simulink model "cooling_system"  (R2025b)
settings: Solver=ode4  StartTime=0.0  StopTime=200  FixedStep=0.1  RelTol=1e-3
libraries: simulink x14
settings Model: Creator=srija  LastModifiedBy=srija

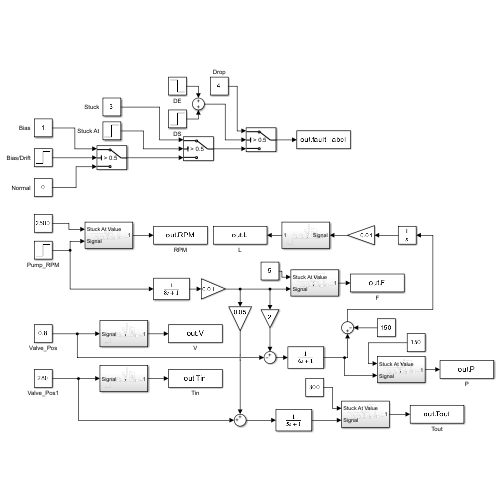
[thumbnail: Simulink's stored preview of the top-level diagram]
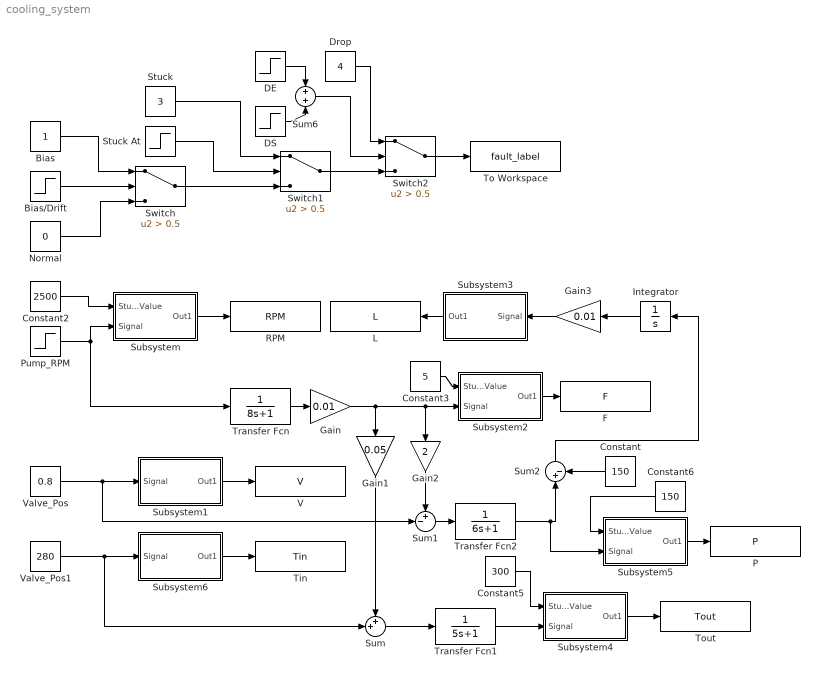
== system cooling_system ==
  Bias : Constant
  Bias/Drift : Step  Time=60  SampleTime=0
  Constant : Constant  Value=150
  Constant2 : Constant  Value=2500
  Constant3 : Constant  Value=5
  Constant5 : Constant  Value=300
  Constant6 : Constant  Value=150
  DE : Step  Time=150  After=-1  SampleTime=0
  DS : Step  Time=140  SampleTime=0
  Drop : Constant  Value=4
  F : ToWorkspace  VariableName=F  SampleTime=-1
  Gain : Gain  Gain=0.01
  Gain1 : Gain  Gain=0.05
  Gain2 : Gain  Gain=2
  Gain3 : Gain  Gain=0.01
  Integrator : Integrator
  L : ToWorkspace  VariableName=L  SampleTime=-1
  Normal : Constant  Value=0
  P : ToWorkspace  VariableName=P  SampleTime=-1
  Pump_RPM : Step  Time=5  Before=1500  After=3000  SampleTime=0
  RPM : ToWorkspace  VariableName=RPM  SampleTime=-1
  Stuck : Constant  Value=3
  Stuck At : Step  Time=120  SampleTime=0
  Subsystem : Subsystem
  Subsystem1 : Subsystem
  Subsystem2 : Subsystem
  Subsystem3 : Subsystem
  Subsystem4 : Subsystem
  Subsystem5 : Subsystem
  Subsystem6 : Subsystem
  Sum : Sum  Inputs=++|
  Sum1 : Sum  Inputs=+-|
  Sum2 : Sum  Inputs=|+-
  Sum6 : Sum  Inputs=+|+
  Switch : Switch  Criteria=u2 > Threshold  Threshold=0.5  SaturateOnIntegerOverflow=off  InputSameDT=off
  Switch1 : Switch  Criteria=u2 > Threshold  Threshold=0.5  SaturateOnIntegerOverflow=off  InputSameDT=off
  Switch2 : Switch  Criteria=u2 > Threshold  Threshold=0.5  SaturateOnIntegerOverflow=off  InputSameDT=off
  Tin : ToWorkspace  VariableName=Tin  SampleTime=-1
  To Workspace : ToWorkspace  VariableName=fault_label  SampleTime=-1
  Tout : ToWorkspace  VariableName=Tout  SampleTime=-1
  Transfer Fcn : TransferFcn  Denominator=[8 1]
  Transfer Fcn1 : TransferFcn  Denominator=[5 1]
  Transfer Fcn2 : TransferFcn  Denominator=[6 1]
  V : ToWorkspace  VariableName=V  SampleTime=-1
  Valve_Pos : Constant  Value=0.8
  Valve_Pos1 : Constant  Value=280
  wires:
  Transfer Fcn/1 -> Gain/1
  Gain/1 -> Subsystem2/2(Signal), Gain2/1, Gain1/1
  Valve_Pos/1 -> Sum1/2, Subsystem1/1(Signal)
  Valve_Pos1/1 -> Sum/2, Subsystem6/1(Signal)
  Gain1/1 -> Sum/1
  Sum/1 -> Transfer Fcn1/1
  Transfer Fcn1/1 -> Subsystem4/2(Signal)
  Gain2/1 -> Sum1/1
  Sum1/1 -> Transfer Fcn2/1
  Transfer Fcn2/1 -> Sum2/1, Subsystem5/2(Signal)
  Integrator/1 -> Gain3/1
  Constant/1 -> Sum2/2
  Sum2/1 -> Integrator/1
  Pump_RPM/1 -> Subsystem/2(Signal), Transfer Fcn/1
  Subsystem/1(Out1) -> RPM/1
  Constant2/1 -> Subsystem/1(Stuck At Value)
  Subsystem2/1(Out1) -> F/1
  Constant3/1 -> Subsystem2/1(Stuck At Value)
  Subsystem4/1(Out1) -> Tout/1
  Constant5/1 -> Subsystem4/1(Stuck At Value)
  Subsystem5/1(Out1) -> P/1
  Constant6/1 -> Subsystem5/1(Stuck At Value)
  Subsystem6/1(Out1) -> Tin/1
  Gain3/1 -> Subsystem3/1(Signal)
  Subsystem3/1(Out1) -> L/1
  Subsystem1/1(Out1) -> V/1
  DE/1 -> Sum6/1
  DS/1 -> Sum6/2
  Bias/Drift/1 -> Switch/2
  Switch/1 -> Switch1/3
  Stuck/1 -> Switch1/1
  Stuck At/1 -> Switch1/2
  Sum6/1 -> Switch2/2
  Switch1/1 -> Switch2/3
  Drop/1 -> Switch2/1
  Switch2/1 -> To Workspace/1
  Bias/1 -> Switch/1
  Normal/1 -> Switch/3

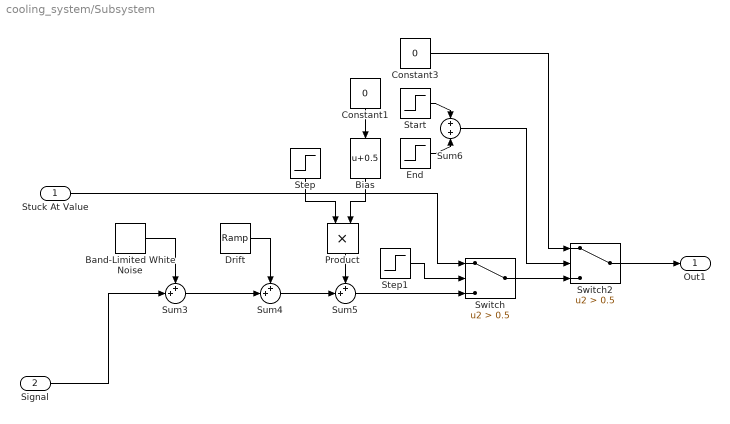
== system cooling_system/Subsystem ==
  Stuck At Value : Inport
  Signal : Inport  Port=2
  Band-Limited White Noise : simulink/Sources/Band-Limited White Noise  Cov=[0.05]  Ts=0.1  seed=[23341]
  Bias : Bias  Bias=0.5  SaturateOnIntegerOverflow=off
  Constant1 : Constant  Value=0
  Constant3 : Constant  Value=0
  Drift : simulink/Sources/Ramp  slope=0.02  start=60  InitialOutput=0
  End : Step  Time=150  After=-1  SampleTime=0
  Product : Product
  Start : Step  Time=140  SampleTime=0
  Step : Step  Time=60  SampleTime=0
  Step1 : Step  Time=120  SampleTime=0
  Sum3 : Sum  Inputs=++|
  Sum4 : Sum  Inputs=++|
  Sum5 : Sum  Inputs=++|
  Sum6 : Sum  Inputs=+|+
  Switch : Switch  Criteria=u2 > Threshold  Threshold=0.5  SaturateOnIntegerOverflow=off  InputSameDT=off
  Switch2 : Switch  Criteria=u2 > Threshold  Threshold=0.5  SaturateOnIntegerOverflow=off  InputSameDT=off
  Out1 : Outport
  wires:
  Drift/1 -> Sum4/1
  Bias/1 -> Product/2
  Sum6/1 -> Switch2/2
  Signal/1 -> Sum3/2
  Product/1 -> Sum5/1
  Sum4/1 -> Sum5/2
  Constant1/1 -> Bias/1
  Band-Limited White Noise/1 -> Sum3/1
  Step/1 -> Product/1
  Step1/1 -> Switch/2
  Sum3/1 -> Sum4/2
  Switch2/1 -> Out1/1
  Constant3/1 -> Switch2/1
  Switch/1 -> Switch2/3
  Start/1 -> Sum6/1
  Stuck At Value/1 -> Switch/1
  End/1 -> Sum6/2
  Sum5/1 -> Switch/3

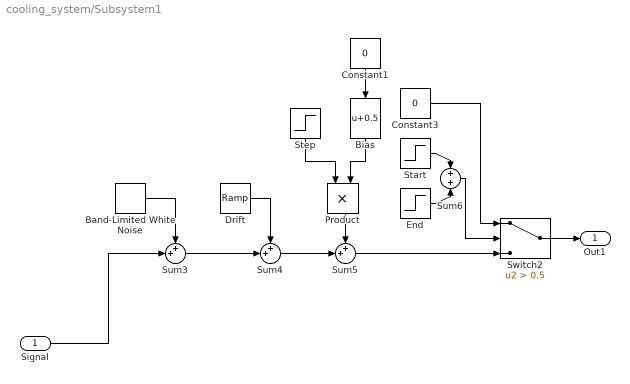
== system cooling_system/Subsystem1 ==
  Signal : Inport
  Band-Limited White Noise : simulink/Sources/Band-Limited White Noise  Cov=[0.05]  Ts=0.1  seed=[23341]
  Bias : Bias  Bias=0.5  SaturateOnIntegerOverflow=off
  Constant1 : Constant  Value=0
  Constant3 : Constant  Value=0
  Drift : simulink/Sources/Ramp  slope=0.02  start=60  InitialOutput=0
  End : Step  Time=150  After=-1  SampleTime=0
  Product : Product
  Start : Step  Time=140  SampleTime=0
  Step : Step  Time=60  SampleTime=0
  Sum3 : Sum  Inputs=++|
  Sum4 : Sum  Inputs=++|
  Sum5 : Sum  Inputs=++|
  Sum6 : Sum  Inputs=+|+
  Switch2 : Switch  Criteria=u2 > Threshold  Threshold=0.5  SaturateOnIntegerOverflow=off  InputSameDT=off
  Out1 : Outport
  wires:
  Sum5/1 -> Switch2/3
  End/1 -> Sum6/2
  Start/1 -> Sum6/1
  Constant3/1 -> Switch2/1
  Switch2/1 -> Out1/1
  Sum3/1 -> Sum4/2
  Step/1 -> Product/1
  Band-Limited White Noise/1 -> Sum3/1
  Constant1/1 -> Bias/1
  Sum4/1 -> Sum5/2
  Product/1 -> Sum5/1
  Signal/1 -> Sum3/2
  Sum6/1 -> Switch2/2
  Bias/1 -> Product/2
  Drift/1 -> Sum4/1

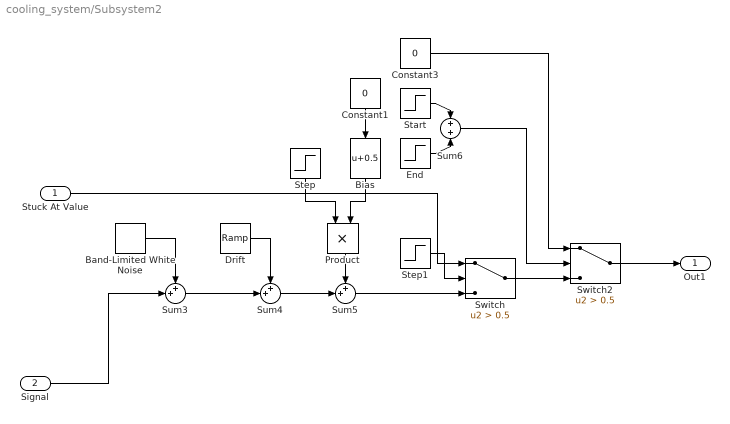
== system cooling_system/Subsystem2 ==
  Stuck At Value : Inport
  Signal : Inport  Port=2
  Band-Limited White Noise : simulink/Sources/Band-Limited White Noise  Cov=[0.05]  Ts=0.1  seed=[23341]
  Bias : Bias  Bias=0.5  SaturateOnIntegerOverflow=off
  Constant1 : Constant  Value=0
  Constant3 : Constant  Value=0
  Drift : simulink/Sources/Ramp  slope=0.02  start=60  InitialOutput=0
  End : Step  Time=150  After=-1  SampleTime=0
  Product : Product
  Start : Step  Time=140  SampleTime=0
  Step : Step  Time=60  SampleTime=0
  Step1 : Step  Time=120  SampleTime=0
  Sum3 : Sum  Inputs=++|
  Sum4 : Sum  Inputs=++|
  Sum5 : Sum  Inputs=++|
  Sum6 : Sum  Inputs=+|+
  Switch : Switch  Criteria=u2 > Threshold  Threshold=0.5  SaturateOnIntegerOverflow=off  InputSameDT=off
  Switch2 : Switch  Criteria=u2 > Threshold  Threshold=0.5  SaturateOnIntegerOverflow=off  InputSameDT=off
  Out1 : Outport
  wires:
  Drift/1 -> Sum4/1
  Bias/1 -> Product/2
  Sum6/1 -> Switch2/2
  Signal/1 -> Sum3/2
  Product/1 -> Sum5/1
  Sum4/1 -> Sum5/2
  Constant1/1 -> Bias/1
  Band-Limited White Noise/1 -> Sum3/1
  Step/1 -> Product/1
  Step1/1 -> Switch/2
  Sum3/1 -> Sum4/2
  Switch2/1 -> Out1/1
  Constant3/1 -> Switch2/1
  Switch/1 -> Switch2/3
  Start/1 -> Sum6/1
  Stuck At Value/1 -> Switch/1
  End/1 -> Sum6/2
  Sum5/1 -> Switch/3

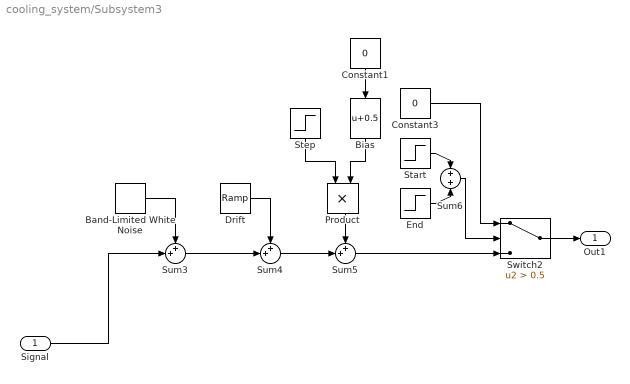
== system cooling_system/Subsystem3 ==
  Signal : Inport
  Band-Limited White Noise : simulink/Sources/Band-Limited White Noise  Cov=[0.05]  Ts=0.1  seed=[23341]
  Bias : Bias  Bias=0.5  SaturateOnIntegerOverflow=off
  Constant1 : Constant  Value=0
  Constant3 : Constant  Value=0
  Drift : simulink/Sources/Ramp  slope=0.02  start=60  InitialOutput=0
  End : Step  Time=150  After=-1  SampleTime=0
  Product : Product
  Start : Step  Time=140  SampleTime=0
  Step : Step  Time=60  SampleTime=0
  Sum3 : Sum  Inputs=++|
  Sum4 : Sum  Inputs=++|
  Sum5 : Sum  Inputs=++|
  Sum6 : Sum  Inputs=+|+
  Switch2 : Switch  Criteria=u2 > Threshold  Threshold=0.5  SaturateOnIntegerOverflow=off  InputSameDT=off
  Out1 : Outport
  wires:
  Sum5/1 -> Switch2/3
  End/1 -> Sum6/2
  Start/1 -> Sum6/1
  Constant3/1 -> Switch2/1
  Switch2/1 -> Out1/1
  Sum3/1 -> Sum4/2
  Step/1 -> Product/1
  Band-Limited White Noise/1 -> Sum3/1
  Constant1/1 -> Bias/1
  Sum4/1 -> Sum5/2
  Product/1 -> Sum5/1
  Signal/1 -> Sum3/2
  Sum6/1 -> Switch2/2
  Bias/1 -> Product/2
  Drift/1 -> Sum4/1

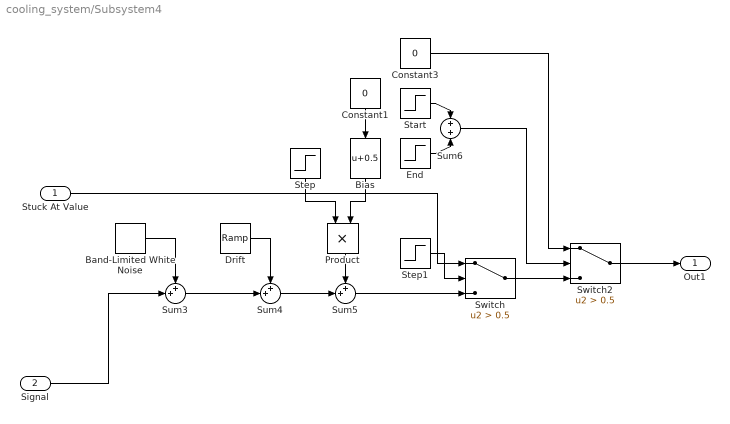
== system cooling_system/Subsystem4 ==
  Stuck At Value : Inport
  Signal : Inport  Port=2
  Band-Limited White Noise : simulink/Sources/Band-Limited White Noise  Cov=[0.05]  Ts=0.1  seed=[23341]
  Bias : Bias  Bias=0.5  SaturateOnIntegerOverflow=off
  Constant1 : Constant  Value=0
  Constant3 : Constant  Value=0
  Drift : simulink/Sources/Ramp  slope=0.02  start=60  InitialOutput=0
  End : Step  Time=150  After=-1  SampleTime=0
  Product : Product
  Start : Step  Time=140  SampleTime=0
  Step : Step  Time=60  SampleTime=0
  Step1 : Step  Time=120  SampleTime=0
  Sum3 : Sum  Inputs=++|
  Sum4 : Sum  Inputs=++|
  Sum5 : Sum  Inputs=++|
  Sum6 : Sum  Inputs=+|+
  Switch : Switch  Criteria=u2 > Threshold  Threshold=0.5  SaturateOnIntegerOverflow=off  InputSameDT=off
  Switch2 : Switch  Criteria=u2 > Threshold  Threshold=0.5  SaturateOnIntegerOverflow=off  InputSameDT=off
  Out1 : Outport
  wires:
  Drift/1 -> Sum4/1
  Bias/1 -> Product/2
  Sum6/1 -> Switch2/2
  Signal/1 -> Sum3/2
  Product/1 -> Sum5/1
  Sum4/1 -> Sum5/2
  Constant1/1 -> Bias/1
  Band-Limited White Noise/1 -> Sum3/1
  Step/1 -> Product/1
  Step1/1 -> Switch/2
  Sum3/1 -> Sum4/2
  Switch2/1 -> Out1/1
  Constant3/1 -> Switch2/1
  Switch/1 -> Switch2/3
  Start/1 -> Sum6/1
  Stuck At Value/1 -> Switch/1
  End/1 -> Sum6/2
  Sum5/1 -> Switch/3

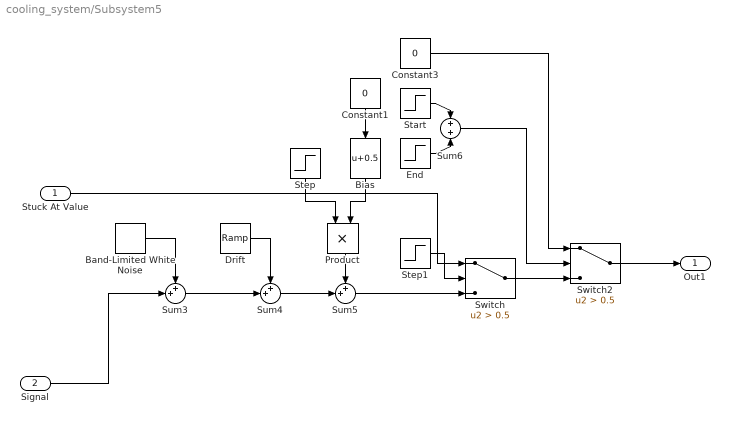
== system cooling_system/Subsystem5 ==
  Stuck At Value : Inport
  Signal : Inport  Port=2
  Band-Limited White Noise : simulink/Sources/Band-Limited White Noise  Cov=[0.05]  Ts=0.1  seed=[23341]
  Bias : Bias  Bias=0.5  SaturateOnIntegerOverflow=off
  Constant1 : Constant  Value=0
  Constant3 : Constant  Value=0
  Drift : simulink/Sources/Ramp  slope=0.02  start=60  InitialOutput=0
  End : Step  Time=150  After=-1  SampleTime=0
  Product : Product
  Start : Step  Time=140  SampleTime=0
  Step : Step  Time=60  SampleTime=0
  Step1 : Step  Time=120  SampleTime=0
  Sum3 : Sum  Inputs=++|
  Sum4 : Sum  Inputs=++|
  Sum5 : Sum  Inputs=++|
  Sum6 : Sum  Inputs=+|+
  Switch : Switch  Criteria=u2 > Threshold  Threshold=0.5  SaturateOnIntegerOverflow=off  InputSameDT=off
  Switch2 : Switch  Criteria=u2 > Threshold  Threshold=0.5  SaturateOnIntegerOverflow=off  InputSameDT=off
  Out1 : Outport
  wires:
  Sum5/1 -> Switch/3
  End/1 -> Sum6/2
  Stuck At Value/1 -> Switch/1
  Start/1 -> Sum6/1
  Switch/1 -> Switch2/3
  Constant3/1 -> Switch2/1
  Switch2/1 -> Out1/1
  Sum3/1 -> Sum4/2
  Step1/1 -> Switch/2
  Step/1 -> Product/1
  Band-Limited White Noise/1 -> Sum3/1
  Constant1/1 -> Bias/1
  Sum4/1 -> Sum5/2
  Product/1 -> Sum5/1
  Signal/1 -> Sum3/2
  Sum6/1 -> Switch2/2
  Bias/1 -> Product/2
  Drift/1 -> Sum4/1

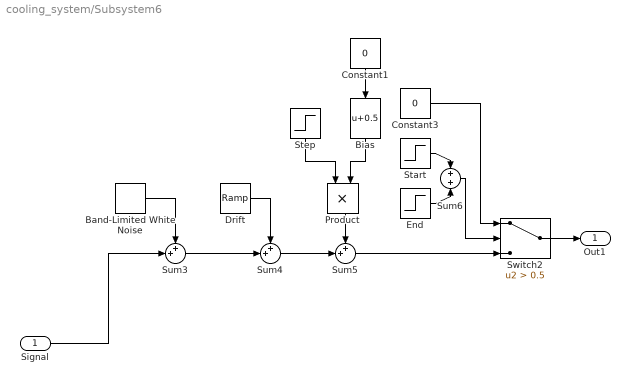
== system cooling_system/Subsystem6 ==
  Signal : Inport
  Band-Limited White Noise : simulink/Sources/Band-Limited White Noise  Cov=[0.05]  Ts=0.1  seed=[23341]
  Bias : Bias  Bias=0.5  SaturateOnIntegerOverflow=off
  Constant1 : Constant  Value=0
  Constant3 : Constant  Value=0
  Drift : simulink/Sources/Ramp  slope=0.02  start=60  InitialOutput=0
  End : Step  Time=150  After=-1  SampleTime=0
  Product : Product
  Start : Step  Time=140  SampleTime=0
  Step : Step  Time=60  SampleTime=0
  Sum3 : Sum  Inputs=++|
  Sum4 : Sum  Inputs=++|
  Sum5 : Sum  Inputs=++|
  Sum6 : Sum  Inputs=+|+
  Switch2 : Switch  Criteria=u2 > Threshold  Threshold=0.5  SaturateOnIntegerOverflow=off  InputSameDT=off
  Out1 : Outport
  wires:
  Drift/1 -> Sum4/1
  Bias/1 -> Product/2
  Sum6/1 -> Switch2/2
  Signal/1 -> Sum3/2
  Product/1 -> Sum5/1
  Sum4/1 -> Sum5/2
  Constant1/1 -> Bias/1
  Band-Limited White Noise/1 -> Sum3/1
  Step/1 -> Product/1
  Sum3/1 -> Sum4/2
  Switch2/1 -> Out1/1
  Constant3/1 -> Switch2/1
  Start/1 -> Sum6/1
  End/1 -> Sum6/2
  Sum5/1 -> Switch2/3
